simulink library "localApparentWind_ul"  (R2020a)
settings: Solver=VariableStepAuto  StartTime=0.0  StopTime=10.0  RelTol=1e-3
libraries: vrlib x1
settings Model: Creator=mcobb  LastModifiedBy=John Jr
settings DataIOCC: ReturnWorkspaceOutputs=off
settings DebuggingCC: ArithmeticOperatorsInVariantConditions=warning
settings SFSimCC: CustomCodeUndefinedFunction=UseInterfaceOnly

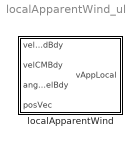
== system localApparentWind_ul ==
  localApparentWind : Subsystem

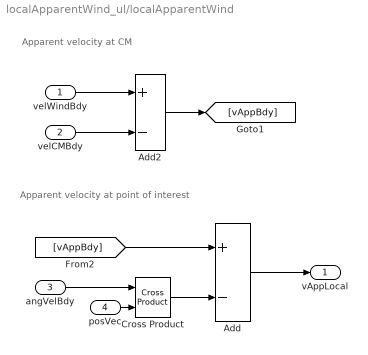
== system localApparentWind_ul/localApparentWind ==
  note: Apparent velocity at CM
  note: Apparent velocity at point of interest
  velWindBdy : Inport
  velCMBdy : Inport  Port=2
  angVelBdy : Inport  Port=3
  posVec : Inport  Port=4
  Add : Sum  Inputs=+-
  Add2 : Sum  Inputs=+-
  Cross Product : vrlib/Utilities/Cross Product
  vAppLocal : Outport  VectorParamsAs1DForOutWhenUnconnected=off
  wires:
  angVelBdy/1 -> Cross Product/1
  [vAppBdy] -> Add/1
  Add2/1 -> [vAppBdy]
  velCMBdy/1 -> Add2/2
  velWindBdy/1 -> Add2/1
  Cross Product/1 -> Add/2
  posVec/1 -> Cross Product/2
  Add/1 -> vAppLocal/1
